simulink model "test1"  (R2021a)
settings: Solver=ode45  StartTime=0.0  StopTime=timestop  RelTol=1e-3
values from neighbouring files (symbols this model uses):
  a = a_1M    [MODEL_OUTPUT.m]    (also in test1_script.m = 10)
  g = g_1M    [MODEL_OUTPUT.m]    (also in test1_script.m = 1)
  k = k_1M    [MODEL_OUTPUT.m]    (also in test1_script.m = 0.1)
  x0 = 1    [test1_script.m]
  y0 = 0.01    [test1_script.m]
libraries: simulink x3, aerolibanim x1
settings Model: Creator=vanya  LastModifiedBy=vanya
settings SolverCC: ZeroCrossControl=DisableAll

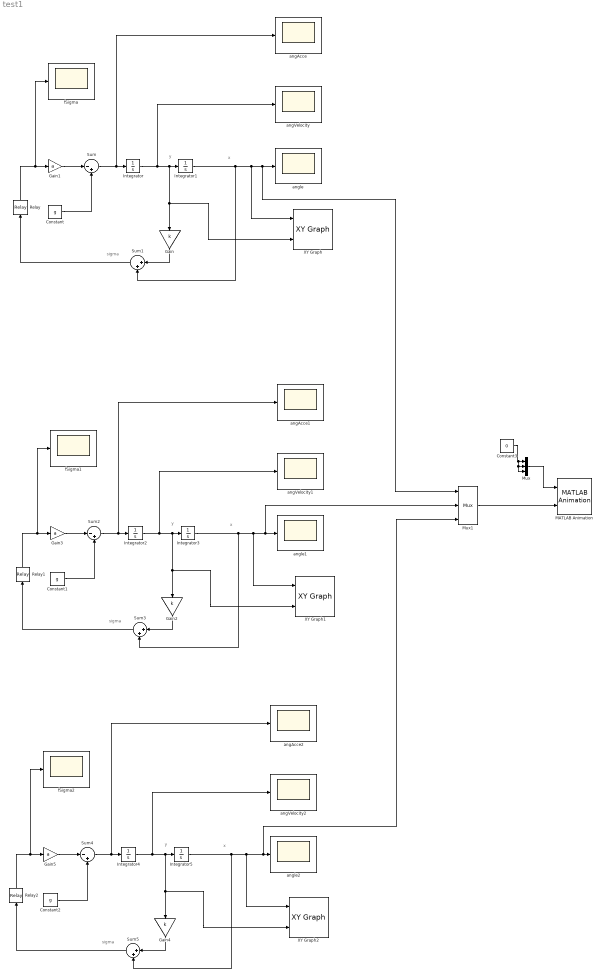
== system test1 ==
  note: sigma
  note: y
  note: x
  note: sigma
  note: x
  note: y
  note: sigma
  note: x
  note: y
  Constant : Constant  Value=g
  Constant1 : Constant  Value=g
  Constant2 : Constant  Value=g
  Constant3 : Constant  Value=0
  Gain : Gain  Gain=k
  Gain1 : Gain  Gain=a
  Gain2 : Gain  Gain=k
  Gain3 : Gain  Gain=a
  Gain4 : Gain  Gain=k
  Gain5 : Gain  Gain=a
  Integrator : Integrator  InitialCondition=y0
  Integrator1 : Integrator  InitialCondition=x0
  Integrator2 : Integrator  InitialCondition=y0
  Integrator3 : Integrator  InitialCondition=x0
  Integrator4 : Integrator  InitialCondition=y0
  Integrator5 : Integrator  InitialCondition=x0
  MATLAB Animation : aerolibanim/MATLAB Animation  Tag=Matlab Animation 6 DOF  Vehicles=1  Geometries='astredwedge.mat'  BoundingBoxCoordinates=[-50,50,-50,50,-50,50]  CameraOffset=[50,50,50]  CameraViewAngle=3  SampleTime=0.2  FigurePosition=[1243,487,498,345]
      settings: SourceProductBaseCode=AE
  Mux : Mux  Inputs=3
  Mux1 : Mux  Inputs=3
  Relay : Relay  OnSwitchValue=0  OffSwitchValue=0  OffOutputValue=-1
  Relay1 : Relay  OnSwitchValue=0  OffSwitchValue=0  OffOutputValue=-1
  Relay2 : Relay  OnSwitchValue=0  OffSwitchValue=0  OffOutputValue=-1
  Sum : Sum  Inputs=|-+
  Sum1 : Sum  Inputs=|++
  Sum2 : Sum  Inputs=|-+
  Sum3 : Sum  Inputs=|++
  Sum4 : Sum  Inputs=|-+
  Sum5 : Sum  Inputs=|++
  XY Graph : simulink/Sinks/XY Graph  xmin=-2  xmax=2  ymin=-4  ymax=3  st=-1
  XY Graph1 : simulink/Sinks/XY Graph  xmin=-2  xmax=2  ymin=-4  ymax=3  st=-1
  XY Graph2 : simulink/Sinks/XY Graph  xmin=-2  xmax=2  ymin=-4  ymax=3  st=-1
  angAcce : Scope
  angAcce1 : Scope
  angAcce2 : Scope
  angVelocity : Scope
  angVelocity1 : Scope
  angVelocity2 : Scope
  angle : Scope
  angle1 : Scope
  angle2 : Scope
  fSigma : Scope
  fSigma1 : Scope
  fSigma2 : Scope
  wires:
  Constant/1 -> Sum/2
  Gain1/1 -> Sum/1
  Sum/1 -> angAcce/1, Integrator/1
  Integrator/1 -> XY Graph/2, Gain/1, Integrator1/1, angVelocity/1
  Integrator1/1 -> Sum1/2, XY Graph/1, Mux1/1, angle/1
  Gain/1 -> Sum1/1
  Sum1/1 -> Relay/1
  Relay/1 -> fSigma/1, Gain1/1
  Relay1/1 -> fSigma1/1, Gain3/1
  Sum2/1 -> angAcce1/1, Integrator2/1
  Integrator2/1 -> XY Graph1/2, Gain2/1, Integrator3/1, angVelocity1/1
  Gain2/1 -> Sum3/1
  Constant1/1 -> Sum2/2
  Gain3/1 -> Sum2/1
  Integrator3/1 -> Sum3/2, XY Graph1/1, Mux1/2, angle1/1
  Sum3/1 -> Relay1/1
  Relay2/1 -> fSigma2/1, Gain5/1
  Sum4/1 -> angAcce2/1, Integrator4/1
  Integrator4/1 -> XY Graph2/2, Gain4/1, Integrator5/1, angVelocity2/1
  Gain4/1 -> Sum5/1
  Constant2/1 -> Sum4/2
  Gain5/1 -> Sum4/1
  Integrator5/1 -> Sum5/2, XY Graph2/1, Mux1/3, angle2/1
  Sum5/1 -> Relay2/1
  Constant3/1 -> Mux/3, Mux/2, Mux/1
  Mux/1 -> MATLAB Animation/1
  Mux1/1 -> MATLAB Animation/2
